simulink model "SubState2SubState_2020a"  (R2020a)
settings: Solver=VariableStepAuto  StartTime=0.0  StopTime=10.0  RelTol=1e-3
settings Model: Creator=apple  LastModifiedBy=apple

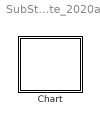
== system SubState2SubState_2020a ==
  Chart : Stateflow chart  TreatAsAtomicUnit=on

== stateflow chart SubState2SubState_2020a/Chart ==
  state A
    en:fprintf("entryA");
    du:fprintf("duringA");
    ex:fprintf("exitA");
    state A2
    state A1
      en:fprintf("entryA1");
      du:fprintf("duringA1");
      ex:fprintf("exitA1");
    (default) -> A1
  state B
    en:fprintf("entryB");
    du:fprintf("duringB");
    ex:fprintf("exitB");
    state B2
    state B1
      en:fprintf("entryB1");
      du:fprintf("duringB1");
      ex:fprintf("exitB1");
    (default) -> B1
  (default) -> A
  A1 -> B1 : E_one/{fprintf("transition_action")}
  events: E_one local FUNCTION_CALL_EVENT
